simulink model "model2"  (R2019a)
settings: Solver=ode4  StartTime=0.0  StopTime=0.1  FixedStep=0.001  RelTol=1e-3
values from neighbouring files (symbols this model uses):
  A = [a12*X(3), a11, a12*X(1) ... (first row only)    [lab4.m]
  B = [a13 0 ... (first row only)    [lab4.m]
  Mc = 0.3    [lab4.m]
  Uc = 0    [lab4.m]
  x0 = [0,0,0]    [lab4.m]
settings Model: Creator=Andrew  LastModifiedBy=ogure

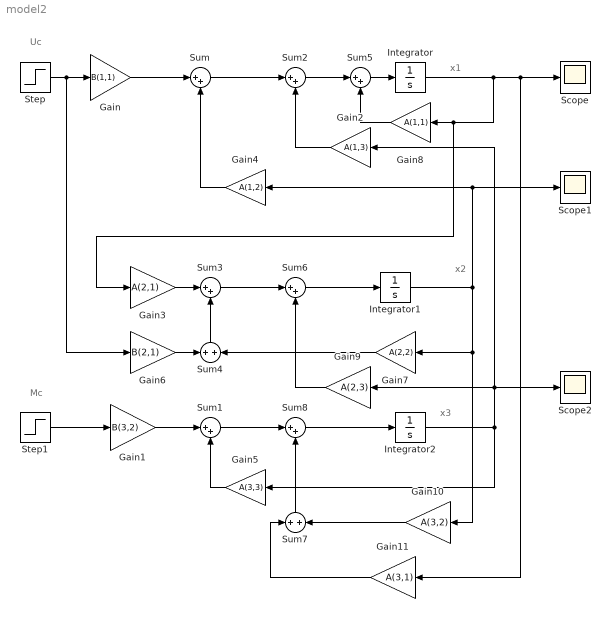
== system model2 ==
  note: x2
  note: Uc
  note: x3
  note: Mc
  note: x1
  Gain : Gain  Gain=B(1,1)
  Gain1 : Gain  Gain=B(3,2)
  Gain10 : Gain  Gain=A(3,2)
  Gain11 : Gain  Gain=A(3,1)
  Gain2 : Gain  Gain=A(1,3)
  Gain3 : Gain  Gain=A(2,1)
  Gain4 : Gain  Gain=A(1,2)
  Gain5 : Gain  Gain=A(3,3)
  Gain6 : Gain  Gain=B(2,1)
  Gain7 : Gain  Gain=A(2,2)
  Gain8 : Gain  Gain=A(1,1)
  Gain9 : Gain  Gain=A(2,3)
  Integrator : Integrator  InitialCondition=x0(1)
  Integrator1 : Integrator  InitialCondition=x0(2)
  Integrator2 : Integrator  InitialCondition=x0(3)
  Scope : Scope
  Scope1 : Scope
  Scope2 : Scope
  Step : Step  Time=0  After=Uc  SampleTime=0
  Step1 : Step  Time=0  After=Mc  SampleTime=0
  Sum{,1..3,5..6,8} (7 alike) : Sum  Inputs=|++
  Sum4 : Sum  Inputs=+|+
  Sum7 : Sum  Inputs=+|+
  wires:
  Gain4/1 -> Sum/2
  Gain1/1 -> Sum1/1
  Gain5/1 -> Sum1/2
  Integrator/1 -> Gain3/1, Gain8/1, Gain11/1, Scope/1
  Gain/1 -> Sum/1
  Sum/1 -> Sum2/1
  Step1/1 -> Gain1/1
  Gain2/1 -> Sum2/2
  Sum3/1 -> Sum6/1
  Integrator1/1 -> Gain4/1, Scope1/1, Gain10/1, Gain7/1
  Gain6/1 -> Sum4/1
  Step/1 -> Gain6/1, Gain/1
  Gain7/1 -> Sum4/2
  Sum4/1 -> Sum3/2
  Gain3/1 -> Sum3/1
  Integrator2/1 -> Gain2/1, Scope2/1, Gain9/1, Gain5/1
  Sum5/1 -> Integrator/1
  Sum2/1 -> Sum5/1
  Gain8/1 -> Sum5/2
  Gain9/1 -> Sum6/2
  Sum6/1 -> Integrator1/1
  Gain11/1 -> Sum7/1
  Gain10/1 -> Sum7/2
  Sum1/1 -> Sum8/1
  Sum7/1 -> Sum8/2
  Sum8/1 -> Integrator2/1
